simulink model "SendUdp2Kinarm"  (R2022a)
settings: Solver=VariableStepAuto  StartTime=0.0  StopTime=10.0  RelTol=1e-3
libraries: slrealtimeiplib x4, slrealtimeutilitieslib x2
settings Model: Creator=willy  LastModifiedBy=Willy Lee
settings DebuggingCC: UnconnectedInputMsg=warning  UnconnectedOutputMsg=warning  UnconnectedLineMsg=warning
settings RTWCC: DLArmComputeVersion=19.05

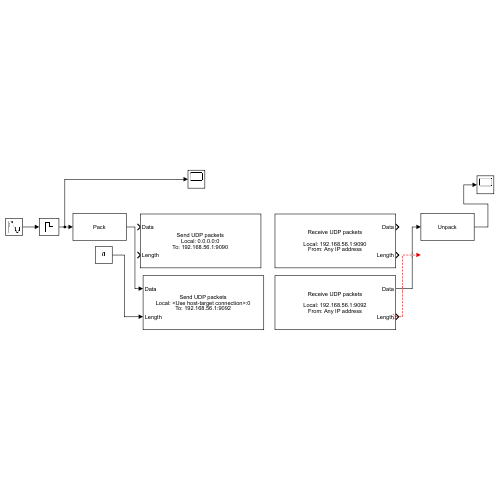
[thumbnail: Simulink's stored preview of the top-level diagram]
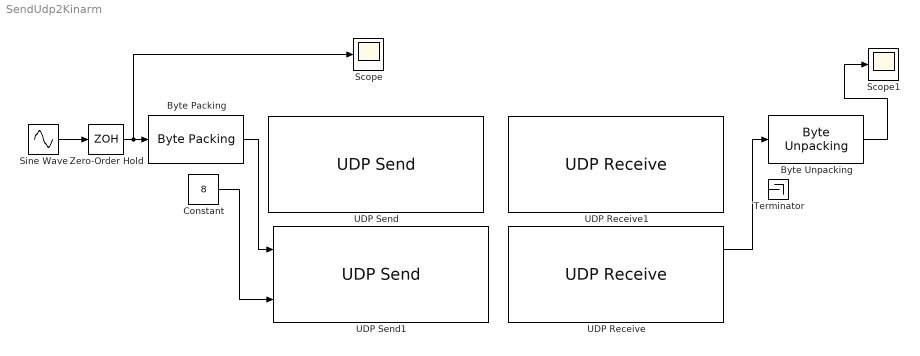
== system SendUdp2Kinarm ==
  Byte Packing : slrealtimeutilitieslib/Byte Packing  MaskPackedDataType=uint8  MaskUnpackedDataTypes={'double'}  MaskAlignment=1
  Byte Unpacking : slrealtimeutilitieslib/Byte Unpacking  MaskUnpackedDataTypes={'double'}  MaskUnpackedDataSizes={[1]}  MaskAlignment=1
      settings: SourceProductBaseCode=XP
  Constant : Constant  Value=8  SampleTime=0.01
  Scope : Scope
  Scope1 : Scope
  Sine Wave : Sin  SampleTime=0.01
  Terminator : Terminator
  UDP Receive : slrealtimeiplib/UDP Receive  useHostTargetConn=off  ipAddress=192.168.56.1  localPort=9092  rcvWidth=8  rcvFmAny=on  fmAddress='10.10.10.10'  sampleTime=0.01  enableMessage=off  maxPackets=1
      settings: SourceProductBaseCode=XP
  UDP Receive1 : slrealtimeiplib/UDP Receive  useHostTargetConn=off  ipAddress=192.168.56.1  localPort=9090  rcvWidth=8  rcvFmAny=on  fmAddress='10.10.10.10'  sampleTime=0.01  enableMessage=off  maxPackets=1
      settings: SourceProductBaseCode=XP
  UDP Send : slrealtimeiplib/UDP Send  useHostTargetConn=off  toAddress=192.168.56.1  toPort=9090  sampleTime=0.01  enableMessage=off
      settings: SourceProductBaseCode=XP
  UDP Send1 : slrealtimeiplib/UDP Send  useHostTargetConn=on  toAddress=192.168.56.1  toPort=9092  sampleTime=0.01  enableMessage=off
      settings: SourceProductBaseCode=XP
  Zero-Order Hold : ZeroOrderHold  SampleTime=-1
  wires:
  Zero-Order Hold/1 -> Scope/1, Byte Packing/1
  Sine Wave/1 -> Zero-Order Hold/1
  Byte Unpacking/1 -> Scope1/1
  UDP Receive/1 -> Byte Unpacking/1
  ? -> Terminator/1
  Byte Packing/1 -> UDP Send1/1
  Constant/1 -> UDP Send1/2
